simulink model "general_Test"  (R2022a)
settings: Solver=VariableStepAuto  StartTime=0.0  StopTime=10.0  RelTol=1e-3
settings Model: Creator=umber  LastModifiedBy=umber
settings DataIOCC: ExternalInput=a.getElement('current')  LoadExternalInput=on

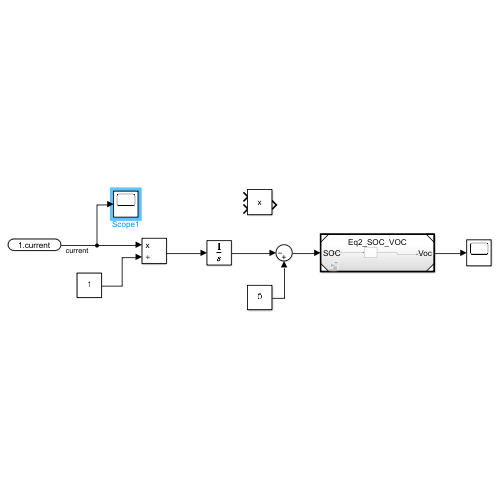
[thumbnail: Simulink's stored preview of the top-level diagram]
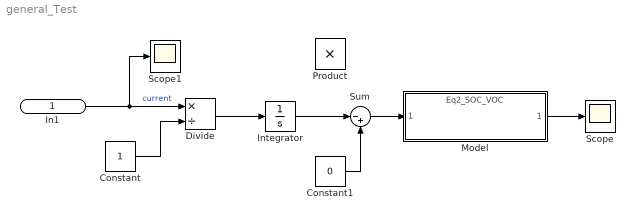
== system general_Test ==
  In1 : Inport
  Constant : Constant
  Constant1 : Constant  Value=0
  Divide : Product  Inputs=*/
  Integrator : Integrator
  Model : ModelReference  ModelNameDialog=Eq2_SOC_VOC.slx  SimulationMode=Normal  ModelReferenceVersion=1.2
  Product : Product
  Scope : Scope
  Scope1 : Scope
  Sum : Sum  Inputs=|-+
  wires:
  Divide/1 -> Integrator/1
  Integrator/1 -> Sum/1
  Sum/1 -> Model/1
  In1/1 -> Scope1/1, Divide/1  "current"
  Constant/1 -> Divide/2
  Constant1/1 -> Sum/2
  Model/1 -> Scope/1
